simulink model "batsolarcomb3"  (R2024b)
settings: Solver=ode45  StartTime=0.0  StopTime=1  RelTol=1e-3  EnableMultiTasking=on
undefined symbols (not defined in the file): Ion, Lithium
libraries: spsSeriesRLCBranchLib x8, spsCurrentMeasurementLib x4, spsMosfetLib x3, spsDiodeLib x2, simulink_need_slupdate x2, simulink x2, spsVoltageMeasurementLib x2, spsBatteryLib x1, spsIdealSwitchLib x1, spspowerguiLib x1, spsControlledCurrentSourceLib x1
settings Model: Creator=user 1  LastModifiedBy=sonus
settings SolverCC: AlgebraicLoopSolver=TrustRegion
settings DataIOCC: LimitDataPoints=on  SaveFormat=Array  SignalLoggingSaveFormat=ModelDataLogs  ReturnWorkspaceOutputs=off
settings OptimizationCC: ExpressionDepthLimit=2147483647  LifeSpan=inf
settings DebuggingCC: UnderspecifiedInitializationDetection=Classic  MergeDetectMultiDrivingBlocksExec=none  SolverPrmCheckMsg=warning  FcnCallInpInsideContextMsg=warning  UnconnectedInputMsg=warning  UnconnectedOutputMsg=warning  UnconnectedLineMsg=warning  StateNameClashWarn=warning  SFUnexpectedBacktrackingDiag=warning  SFNoUnconditionalDefaultTransitionDiag=warning  SFExecutionAtInitializationDiag=none  ArithmeticOperatorsInVariantConditions=warning
settings HardwareCC: ProdBitPerPointer=32  ProdBitPerSizeT=32  ProdBitPerPtrDiffT=32  ProdLargestAtomicFloat=None  ProdIntDivRoundTo=Undefined  ProdEndianess=Unspecified  ProdWordSize=32  ProdHWDeviceType=32-bit Generic
settings ModelReferenceCC: PropagateSignalLabelsOutOfModel=off
settings SFSimCC: SimUseLocalCustomCode=off  CustomCodeUndefinedFunction=UseInterfaceOnly
settings RTWCC: RTWUseLocalCustomCode=off  GPUComputeCapability=3.5
settings CodeAppCC: StateflowObjectComments=on
settings GRTTargetCC: TargetLangStandard=C89/C90 (ANSI)  CombineOutputUpdateFcns=off  GRTInterface=on
settings ConfigComp: CovMetricSettings=dw  CovSaveCumulativeToWorkspaceVar=on  CovSaveSingleToWorkspaceVar=on  CovExternalEMLEnable=off
settings SimscapeCC: SimscapeNormalizeSystem=off
settings ConfigurationSet: Description=SimMechanics 2G

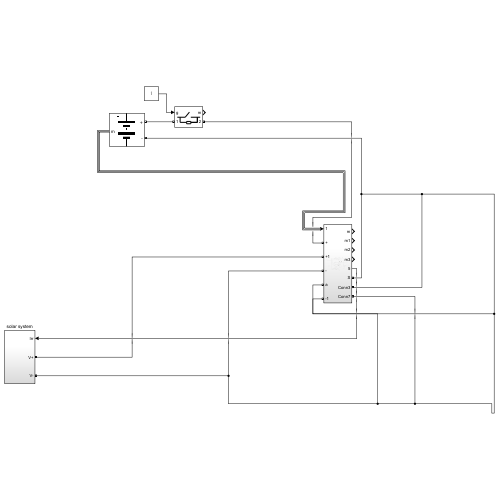
[thumbnail: Simulink's stored preview of the top-level diagram]
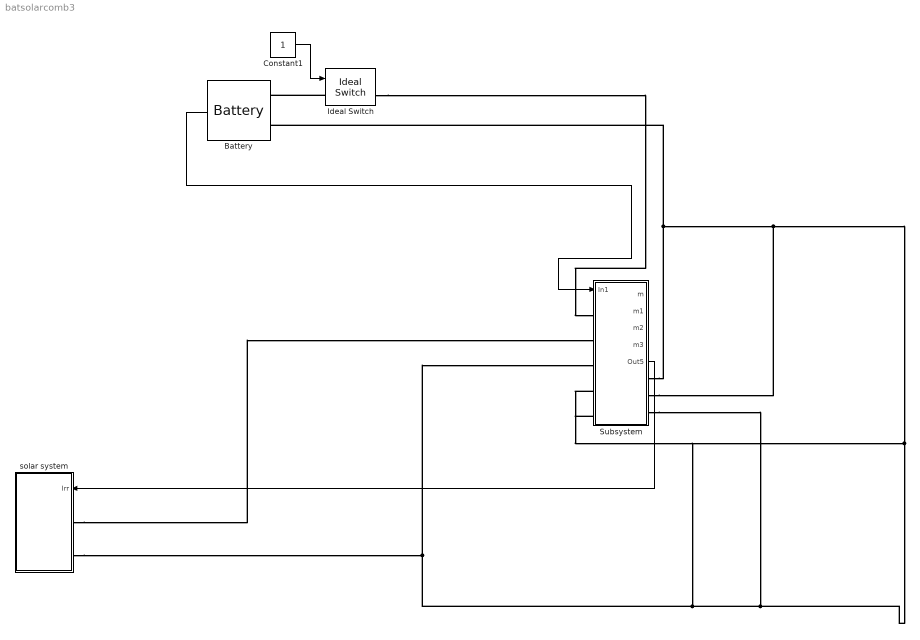
== system batsolarcomb3 ==
  Battery : spsBatteryLib/Battery  BatType=Lithium-Ion  NomV=12  NomQ=6.5  SOC=50  Batt_Tr=30  PresetModel=on  MaxQ=6.5  MinV=9  FullV=13.9678  Dis_rate=2.8261  R=0.018462  Normal_OP=5.8783  expZone="[12.9646     0.319348]"
      settings: LibrarySourceBlock=electricdrivelib/Extra Sources/Battery
  Constant1 : Constant
  Ideal Switch : spsIdealSwitchLib/Ideal Switch  Ron=0.001  Lon=0  IC=0  Rs=1e5  Cs=inf  Measurements=on
  Subsystem : Subsystem
  solar system : Subsystem
  wires:
  Constant1/1 -> Ideal Switch/1
  Battery/1 -> Subsystem/1(In1)
  Subsystem/5(Out5) -> solar system/1(Irr)
  connections:
  Ideal Switch/LConn1 -- Battery/LConn1
  solar system/LConn2 -- Subsystem/LConn4 -- Subsystem/LConn5 -- Subsystem/RConn2 -- Subsystem/RConn1 -- Battery/LConn2 -- Subsystem/RConn3 -- Subsystem/LConn3
  Ideal Switch/RConn1 -- Subsystem/LConn1
  solar system/LConn1 -- Subsystem/LConn2

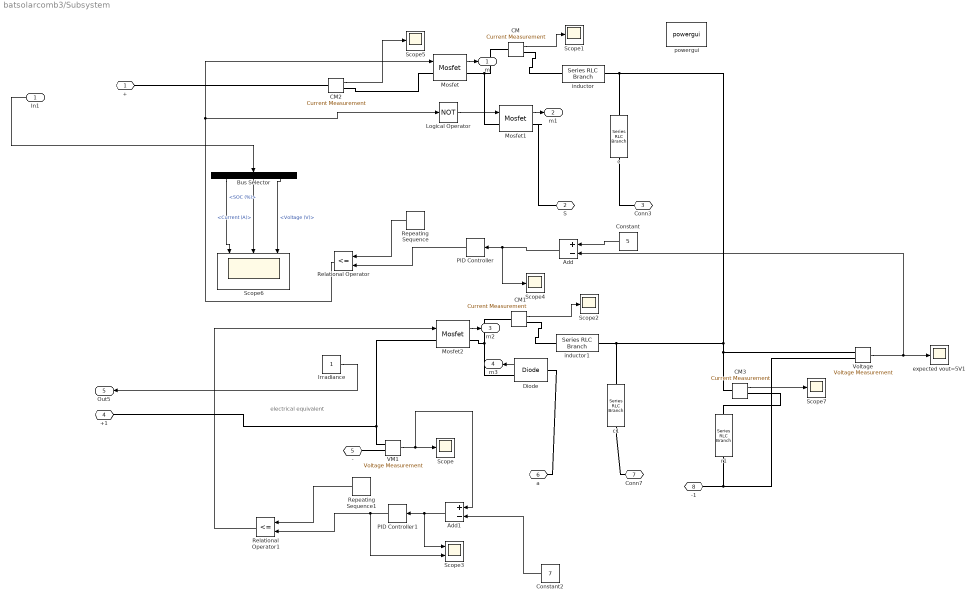
== system batsolarcomb3/Subsystem ==
  note: electrical
      | equivalent
  In1 : Inport
  Add : Sum  Inputs=+-
  Add1 : Sum  Inputs=+-
  Bus Selector : BusSelector  OutputSignals=SOC (%),Current (A),Voltage (V)
  CM{,1..3} (4 alike) : spsCurrentMeasurementLib/Current Measurement  PhasorSimulation=off  OutputType=Complex  PSBequivalent=0
  Constant : Constant  Value=5
  Constant2 : Constant  Value=7
  Diode : spsDiodeLib/Diode  Ron=0.001  Lon=0  Vf=0.8  IC=0  UseSnubber=off  Rs=500  Cs=250e-9  Measurements=on
  Irradiance : Constant
  Logical Operator : Logic  Operator=NOT  AllPortsSameDT=off  OutDataTypeStr=boolean
  Mosfet : spsMosfetLib/Mosfet  Ron=0.1  Lon=0  Rd=0.01  Vfd=0  IC=0  Rs=1e5  Cs=inf  Measurements=on
  Mosfet1 : spsMosfetLib/Mosfet  Ron=0.1  Lon=0  Rd=0.01  Vfd=0  IC=0  Rs=1e5  Cs=inf  Measurements=on
  Mosfet2 : spsMosfetLib/Mosfet  Ron=0.1  Lon=0  Rd=0.01  Vfd=0  IC=0  Rs=1e5  Cs=inf  Measurements=on
  PID Controller : simulink_need_slupdate/PID Controller  P=1  I=5  D=0
  PID Controller1 : simulink_need_slupdate/PID Controller  P=1  I=5  D=0
  Relational Operator : RelationalOperator  Operator=<=  OutDataTypeStr=boolean  InputSameDT=off
  Relational Operator1 : RelationalOperator  Operator=<=  OutDataTypeStr=boolean  InputSameDT=off
  Repeating Sequence : simulink/Sources/Repeating Sequence  rep_seq_t=[0 .5/15e3 1/15e3]  rep_seq_y=[0 1 0]
  Repeating Sequence1 : simulink/Sources/Repeating Sequence  rep_seq_t=[0 .5/15e3 1/15e3]  rep_seq_y=[0 1 0]
  Scope{,1..2,4..5,7} (6 alike) : Scope
  Scope3 : Scope  NumInputPorts=2
  Scope6 : Scope  NumInputPorts=3
  VM1 : spsVoltageMeasurementLib/Voltage Measurement  PhasorSimulation=off  OutputType=Complex  PSBequivalent=0
  Voltage : spsVoltageMeasurementLib/Voltage Measurement  PhasorSimulation=off  OutputType=Complex  PSBequivalent=0
  c : spsSeriesRLCBranchLib/Series RLC Branch  LConnTagsString=__new0  RConnTagsString=__new0  BranchType=C  Resistance=1  Inductance=1e-3  SetiL0=off  InitialCurrent=0  Capacitance=160e-6  Setx0=off  InitialVoltage=0  Measurements=None
  c1 : spsSeriesRLCBranchLib/Series RLC Branch  LConnTagsString=__new0  RConnTagsString=__new0  BranchType=C  Resistance=1  Inductance=1e-3  SetiL0=off  InitialCurrent=0  Capacitance=160e-6  Setx0=off  InitialVoltage=0  Measurements=None
  expected vout=5V1 : Scope
  inductor : spsSeriesRLCBranchLib/Series RLC Branch  LConnTagsString=__new0  RConnTagsString=__new0  BranchType=L  Resistance=1  Inductance=3e-3  SetiL0=off  InitialCurrent=0  Capacitance=1e-6  Setx0=off  InitialVoltage=0  Measurements=None
  inductor1 : spsSeriesRLCBranchLib/Series RLC Branch  LConnTagsString=__new0  RConnTagsString=__new0  BranchType=L  Resistance=1  Inductance=3e-3  SetiL0=off  InitialCurrent=0  Capacitance=1e-6  Setx0=off  InitialVoltage=0  Measurements=None
  powergui : spspowerguiLib/powergui  Priority=1  SimulationMode=Discrete  SampleTime=1e-6  frequency=1  Iterations=50  frequencyindice=0  Pbase=100e6  ErrMax=1e-4  UnitsV=kV  UnitsW=MW  buscounter=0  FunctionMessages=off  echomessages=off  EnableUseOfTLC=off  CurrentSourceSwitches=off  DisableSnubberDevices=off  DisableRonSwitches=off  DisableVfSwitches=off  DisplayEquations=off  AutomaticDiscreteSolvers=off  SolverType=Tustin/Backward Euler (TBE)  Interpol=off  ExternalGateDelay=off  methode=off  Ts=100  x0status=blocks  SPID=off  SwTol=0  HookPort=off  NonlinearTolerance=1e-4  nMaxIteration=100  ContinueOnMaxIteration=off  RestoreLinks=warning  ResistiveCurrentMeasurement=off  Frange=[0:2:500]  Ylog=off  Xlog=on  ShowGrid=off  save=off  variable=ZData  structure=0  ZoomFFT=off  StartTime=0.0  cycles=1  DisplayStyle=1  fundamental=60  FreqAxis=off  MaxFrequency=1000  frequencyindicesteady=1  RmsSteady=1  display=off
  r1 : spsSeriesRLCBranchLib/Series RLC Branch  LConnTagsString=__new0  RConnTagsString=__new0  BranchType=R  Resistance=75  Inductance=1e-3  SetiL0=off  InitialCurrent=0  Capacitance=1e-6  Setx0=off  InitialVoltage=0  Measurements=None
  + : PMIOPort  Side=Left
  S : PMIOPort  Port=2  Side=Right
  Conn3 : PMIOPort  Port=3  Side=Right
  +1 : PMIOPort  Port=4  Side=Left
  - : PMIOPort  Port=5  Side=Left
  a : PMIOPort  Port=6  Side=Left
  Conn7 : PMIOPort  Port=7  Side=Right
  -1 : PMIOPort  Port=8  Side=Left
  m : Outport
  m1 : Outport  Port=2
  m2 : Outport  Port=3
  m3 : Outport  Port=4
  Out5 : Outport  Port=5
  wires:
  Bus Selector/3 -> Scope6/3  "<Voltage (V)>"
  Relational Operator/1 -> Mosfet/1, Logical Operator/1
  CM2/1 -> Scope5/1
  Diode/1 -> m3/1
  VM1/1 -> Scope/1, Add1/1
  CM/1 -> Scope1/1
  Voltage/1 -> expected vout=5V1/1, Add/2
  Bus Selector/2 -> Scope6/2  "<Current (A)>"
  Relational Operator1/1 -> Mosfet2/1
  Add/1 -> PID Controller/1, Scope4/1
  Repeating Sequence1/1 -> Relational Operator1/1
  PID Controller1/1 -> Relational Operator1/2, Scope3/2
  Repeating Sequence/1 -> Relational Operator/1
  Constant2/1 -> Add1/2
  Logical Operator/1 -> Mosfet1/1
  Add1/1 -> PID Controller1/1, Scope3/1
  PID Controller/1 -> Relational Operator/2
  Constant/1 -> Add/1
  Bus Selector/1 -> Scope6/1  "<SOC (%)>"
  CM1/1 -> Scope2/1
  CM3/1 -> Scope7/1
  Irradiance/1 -> Out5/1
  In1/1 -> Bus Selector/1
  Mosfet1/1 -> m1/1
  Mosfet2/1 -> m2/1
  Mosfet/1 -> m/1
  connections:
  c/LConn1 -- inductor/RConn1 -- CM3/LConn1 -- Voltage/LConn1 -- inductor1/RConn1 -- c1/LConn1
  CM3/RConn1 -- r1/LConn1
  CM1/RConn1 -- inductor1/LConn1
  +/RConn1 -- CM2/LConn1
  Diode/RConn1 -- Mosfet2/RConn1 -- CM1/LConn1
  Mosfet2/LConn1 -- +1/RConn1 -- VM1/LConn1
  Mosfet1/RConn1 -- S/RConn1
  Mosfet1/LConn1 -- Mosfet/RConn1 -- CM/LConn1
  -/RConn1 -- VM1/LConn2
  c1/RConn1 -- Conn7/RConn1
  CM2/RConn1 -- Mosfet/LConn1
  Voltage/LConn2 -- -1/RConn1 -- r1/RConn1
  CM/RConn1 -- inductor/LConn1
  c/RConn1 -- Conn3/RConn1
  Diode/LConn1 -- a/RConn1

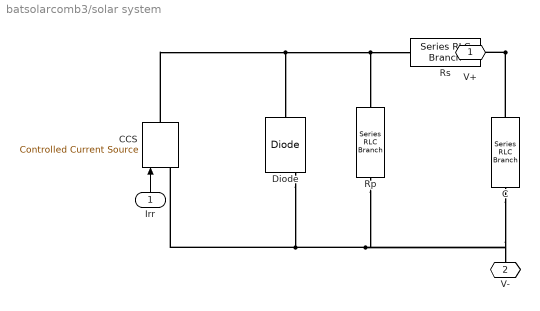
== system batsolarcomb3/solar system ==
  Irr : Inport
  C : spsSeriesRLCBranchLib/Series RLC Branch  LConnTagsString=__new0  RConnTagsString=__new0  BranchType=C  Resistance=0.1  Inductance=1e-3  SetiL0=off  InitialCurrent=0  Capacitance=100e-6  Setx0=off  InitialVoltage=0  Measurements=None
  CCS : spsControlledCurrentSourceLib/Controlled Current Source  Initialize=on  Source_Type=DC  Amplitude=0  Phase=0  Frequency=0  Measurements=None
  Diode : spsDiodeLib/Diode  Ron=0.001  Lon=0  Vf=8.75  IC=0  UseSnubber=off  Rs=500  Cs=250e-9  Measurements=on
  Rp : spsSeriesRLCBranchLib/Series RLC Branch  LConnTagsString=__new0  RConnTagsString=__new0  BranchType=R  Resistance=10000  Inductance=1e-3  SetiL0=off  InitialCurrent=0  Capacitance=1e-6  Setx0=off  InitialVoltage=0  Measurements=None
  Rs : spsSeriesRLCBranchLib/Series RLC Branch  LConnTagsString=__new0  RConnTagsString=__new0  BranchType=R  Resistance=0.1  Inductance=1e-3  SetiL0=off  InitialCurrent=0  Capacitance=1e-6  Setx0=off  InitialVoltage=0  Measurements=None
  V+ : PMIOPort  Side=Left
  V- : PMIOPort  Port=2  Side=Left
  wires:
  Irr/1 -> CCS/1
  connections:
  C/LConn1 -- V+/RConn1 -- Rs/RConn1
  Diode/RConn1 -- Rp/RConn1 -- C/RConn1 -- V-/RConn1 -- CCS/LConn1
  CCS/RConn1 -- Diode/LConn1 -- Rs/LConn1 -- Rp/LConn1
